simulink model "move_Scara"  (Simulink 7.4)
settings: Solver=ode45  StartTime=0.0  StopTime=10.0  RelTol=1e-3
libraries: simulink x1, vrlib x1
settings Model: Creator=filipjuristovski  LastModifiedBy=t6z8
settings DebuggingCC: StrictBusMsg=ErrorLevel1

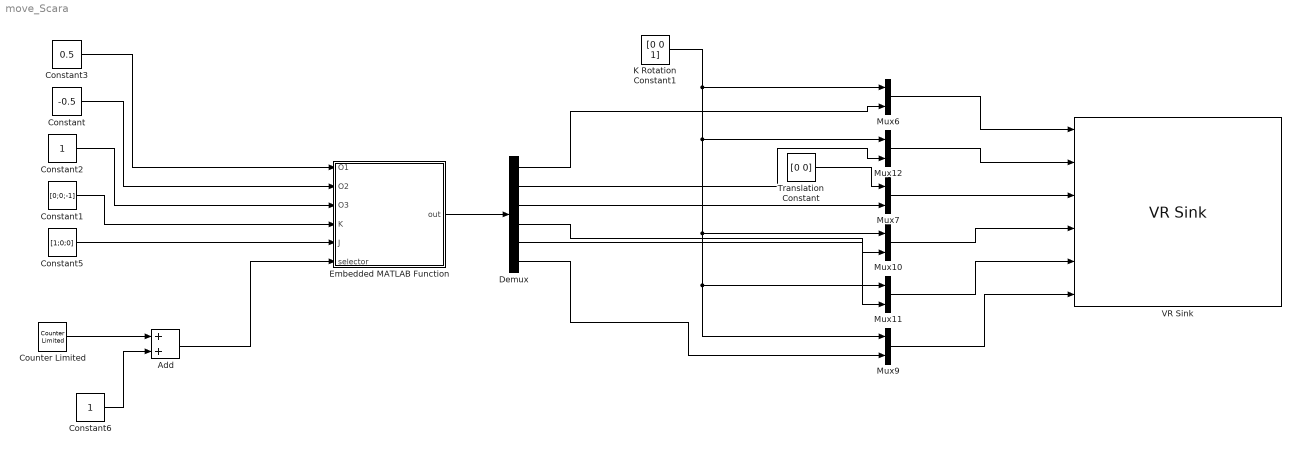
== system move_Scara ==
  Add : Sum  OutDataType=fixdt(1, 16)  OutScaling=2^-10
  Constant : Constant  Value=-0.5  OutDataType=fixdt(1, 16)  OutScaling=2^0
  Constant1 : Constant  Value=[0;0;-1]  VectorParams1D=off  OutDataType=fixdt(1, 16)  OutScaling=2^0
  Constant2 : Constant  OutDataType=fixdt(1, 16)  OutScaling=2^0
  Constant3 : Constant  Value=0.5  OutDataType=fixdt(1, 16)  OutScaling=2^0
  Constant5 : Constant  Value=[1;0;0]  VectorParams1D=off  OutDataType=fixdt(1, 16)  OutScaling=2^0
  Constant6 : Constant  OutDataType=fixdt(1, 16)  OutScaling=2^0
  Counter Limited : simulink/Sources/Counter Limited  SystemSampleTime=-1  uplimit=49  tsamp=-1
  Demux : Demux  Outputs=6
  Embedded MATLAB Function : Stateflow chart  TreatAsAtomicUnit=on
  K Rotation Constant1 : Constant  Value=[0 0 1]
  Mux{6..7,9..12} (6 alike) : Mux  Inputs=2
  Translation Constant : Constant  Value=[0 0]
  VR Sink : vrlib/VR Sink  InstantiateOnLoad=on  SampleTime=-1  ViewEnable=on  RemoteChange=off  RemoteView=on  FieldsWritten=Link_0_Rotation.rotation.4.1.double#Link_1_Rotation.rotation.4.1.double#Link_2_Translation.translation.3.1.double#Link_3_Rotation.rotation.4.1.double#Link_4_Rotation.rotation.4.1.double#Link_5_Rotation.rotation.4.1.double  WorldFileName=SCARAWORLD.WRL  AutoView=off  VideoDimensions=[]
  wires:
  Constant3/1 -> Embedded MATLAB Function/1(O1)
  Constant/1 -> Embedded MATLAB Function/2(O2)
  Constant2/1 -> Embedded MATLAB Function/3(O3)
  Constant1/1 -> Embedded MATLAB Function/4(K)
  Constant5/1 -> Embedded MATLAB Function/5(J)
  K Rotation Constant1/1 -> Mux6/1, Mux10/1, Mux11/1, Mux9/1, Mux12/1
  Translation Constant/1 -> Mux7/1
  Mux6/1 -> VR Sink/1
  Mux12/1 -> VR Sink/2
  Mux7/1 -> VR Sink/3
  Mux10/1 -> VR Sink/4
  Mux11/1 -> VR Sink/5
  Mux9/1 -> VR Sink/6
  Demux/1 -> Mux6/2
  Demux/2 -> Mux12/2
  Demux/3 -> Mux7/2
  Demux/4 -> Mux10/2
  Demux/6 -> Mux9/2
  Demux/5 -> Mux11/2
  Embedded MATLAB Function/1(out) -> Demux/1
  Add/1 -> Embedded MATLAB Function/6(selector)
  Constant6/1 -> Add/2
  Counter Limited/1 -> Add/1

== matlab function Embedded MATLAB Function ==
  data: O1 input double; out output double; O2 input double; O3 input double; K input double; J input double; selector input double
function out  = move_Scara(O1,O2,O3,K,J,selector)
%#eml

T = 1;

CalcPoints = 0:0.02:T;

steps = size(CalcPoints,2);

EndPos = [O1;O2;O3];

%I = cross(J, K);

%EndC6 = [I J K];

% Gripper start coordinates
o6 = [1;1;0];
C6 = [1  0  0;
      0 -1  0;
      0  0 -1];

%rotM = EndC6' * C6;

% Calculate gripper rotation
%rotV = vrrotmat2vec(rotM);

%angle = rotV(4);
%axis = rotV(1:3)';

%angular_v = sin(CalcPoints.*(pi/T));
%angular_v = angular_v .* pi*angle/(2*T);

%ang_v_vectors = axis * angular_v;
  
path = EndPos - o6;

d = norm(path);

% Calculate Velocity
v = sin(CalcPoints.*(pi/T));
v = v .*pi* d/(2*T);

v_vector = path/d;

if d == 0
    v_vector = zeros(3,1);
end

v_vectors = v_vector * v;
qStart = [0; -pi/2; 0; 0; 0; 0];
ang_v_vectors = zeros(size(v_vectors));

q = zeros(size(CalcPoints,2)+1, 6);
qDot = q;
qDotDot = q;

q(1,:) = qStart;

for i = 1:steps
    %Calculate velocity
    jacobian = ScaraJacobian(q(i,:)');
    invJ = pinv(jacobian);
    qDot(i,:) = invJ*[v_vectors(:,i);ang_v_vectors(:,i)];
    
    %qDotDot(i,:) = invJ*(
    
    %Calculate new position
    q(i+1,:) = qDot(i,:)*0.02 + q(i,:);  
end

out = q(selector,:)';
